simulink model "Commande_6_ReglageCascade_LoopShaping"  (R2015a)
settings: Solver=ode45  StartTime=0.0  StopTime=20  RelTol=1e-3
values from neighbouring files (symbols this model uses):
  Kd = p1^2*J4    (= 0.0333)    [A_1_Data.m]    (also in matlab.mat = 0.009)
  Kp = -2*p1*J4    (= 0.00222)    [A_1_Data.m]    (also in matlab.mat = 0.0006)
  s = tf('s')    [A_3_LoopShaping.m]    (also in A_4_Hinfini.m = zpk('s'))
  X = [0;0;0;0;0;0;0;0]    [A_1_Data.m]
  Y = [0;0;0;0;0;0;0;0]    [A_1_Data.m]
undefined symbols (not defined in the file or in its folder): sfun3d, Z
libraries: sm_lib x332, nesl_utility x15, simulink x1
(part 1 of 10)
settings Model: Creator=user  LastModifiedBy=user

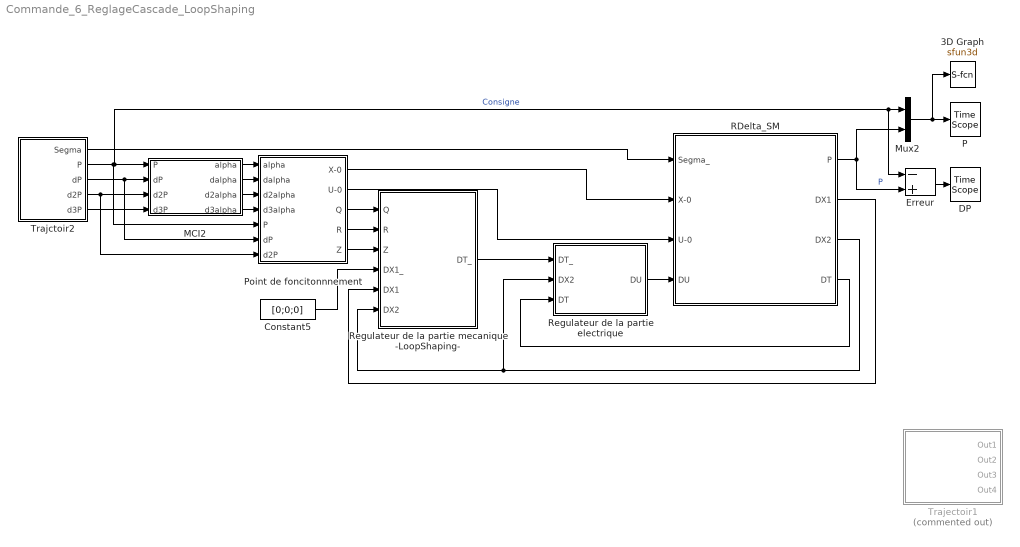
== system Commande_6_ReglageCascade_LoopShaping ==
  3D Graph : S-Function  LoadFcn=sfun3d([],[],[],'LoadBlock')  StartFcn=sfun3d([],[],[],'Start')  StopFcn=sfun3d([],[],[],'Stop')  FunctionName=sfun3d  Parameters=ax,T,np,cp,gd,ls,mk  mask(3D Graph){np=2, ax=[-1 1 -1 1 -2 0]*0.3, cp=[3 2 1], gd=on, ls=-, mk=o, T=0.0001}
      mask prompts: np "Number of point (lines)"; ax "[xmin xmax  ymin ymax zmin zmax]"; cp "Camera position (use [0 0 1] for 2D XY view)"; gd "Grid (on|off)"; ls "LineStyle"; mk "Marker"; T "Sampling Time"
      mask help:
      | This block plots the position of several points in the XYZ space. The input contains the coordinates of all the points (x1,y1,z1,x2,y2,z2,...).
      | The number of points (lines), the XYZ ranges, camera position, grid, linestyle, marker and sampling time, can be set as mask parameters.
      settings: CopyFcn=sfun3d([],[],[],'CopyBlock')  DeleteFcn=sfun3d([],[],[],'DeleteBlock')  NameChangeFcn=sfun3d([],[],[],'NameChange')
      mask Help:
      | This block plots the position of several points in the XYZ space. The input contains the coordinates of all the points (x1,y1,z1,x2,y2,z2,...).
      | The number of points (lines), the XYZ ranges, camera position, grid, linestyle, marker and sampling time, can be set as mask parameters.
      mask TypeOptions ls: - | -- | : | -. | none
      mask TypeOptions mk: none | . | + | o | * | x | square | diamond | v | ^ | > | < | pentagram | hexagram
      mask Display: plot([.05 .95 .95 .05 .05],[.45 .45 .95 .95 .45], 0.5+cos(0:0.1:2*pi)*0.3,0.7+sin(0:0.1:2*pi)*0.2)
  Constant5 : Constant  Value=[0;0;0]
  DP : TimeScope  DefaultConfigurationName=spbscopes.TimeScopeBlockCfg
  Erreur : Sum  Inputs=-+
  MCI2 : MATLAB Function  TreatAsAtomicUnit=on
  Mux2 : Mux  Inputs=2
  P : TimeScope  DefaultConfigurationName=spbscopes.TimeScopeBlockCfg
  Point de foncitonnnement : Subsystem
  RDelta_SM : Subsystem
      mask Display:
      | image(imread('DeltaImage2.PNG'))
      | port_label('input',1,'Segma')
      | port_label('input',2,'X-0')
      | port_label('input',3,'U-0')
      | port_label('input',4,'DU')
      | port_label('output',1,'P')
      | port_label('output',2,'DX1')
      | port_label('output',3,'DX2')
      | port_label('output',4,'DT')
  Regulateur de la partie electrique : Subsystem
  Regulateur de la partie mecanique -LoopShaping- : Subsystem
  Trajctoir2 : Subsystem
  Trajectoir1 : Subsystem  Commented=on
  wires:
  Trajctoir2/2(P) -> Erreur/1, Mux2/1, MCI2/1(P), Point de foncitonnnement/5(P)  "Consigne"
  Trajctoir2/3(dP) -> Point de foncitonnnement/6(dP), MCI2/2(dP)
  Trajctoir2/4(d2P) -> Point de foncitonnnement/7(d2P), MCI2/3(d2P)
  MCI2/3(d2alpha) -> Point de foncitonnnement/3(d2alpha)
  MCI2/2(dalpha) -> Point de foncitonnnement/2(dalpha)
  MCI2/1(alpha) -> Point de foncitonnnement/1(alpha)
  MCI2/4(d3alpha) -> Point de foncitonnnement/4(d3alpha)
  Trajctoir2/5(d3P) -> MCI2/4(d3P)
  RDelta_SM/1(P) -> Mux2/2, Erreur/2  "P"
  Point de foncitonnnement/3(Q) -> Regulateur de la partie mecanique -LoopShaping-/1(Q)
  Point de foncitonnnement/4(R) -> Regulateur de la partie mecanique -LoopShaping-/2(R)
  Point de foncitonnnement/5(Z) -> Regulateur de la partie mecanique -LoopShaping-/3(Z)
  Point de foncitonnnement/2(U-0) -> RDelta_SM/3(U-0)
  Point de foncitonnnement/1(X-0) -> RDelta_SM/2(X-0)
  Regulateur de la partie electrique/1(DU) -> RDelta_SM/4(DU)
  Regulateur de la partie mecanique -LoopShaping-/1(DT_) -> Regulateur de la partie electrique/1(DT_)
  RDelta_SM/4(DT) -> Regulateur de la partie electrique/3(DT)
  RDelta_SM/3(DX2) -> Regulateur de la partie mecanique -LoopShaping-/6(DX2), Regulateur de la partie electrique/2(DX2)
  RDelta_SM/2(DX1) -> Regulateur de la partie mecanique -LoopShaping-/5(DX1)
  Constant5/1 -> Regulateur de la partie mecanique -LoopShaping-/4(DX1_)
  Trajctoir2/1(Segma) -> RDelta_SM/1(Segma_)
  Mux2/1 -> 3D Graph/1, P/1
  Erreur/1 -> DP/1

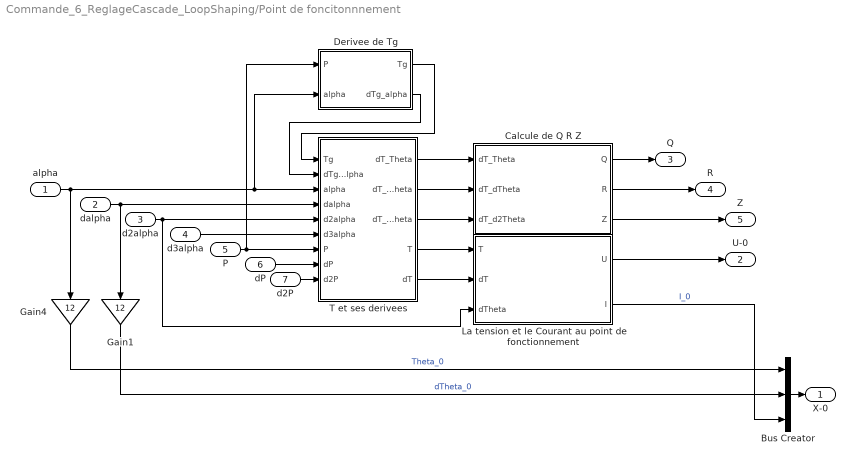
== system Commande_6_ReglageCascade_LoopShaping/Point de foncitonnnement ==
  alpha : Inport
  dalpha : Inport  Port=2
  d2alpha : Inport  Port=3
  d3alpha : Inport  Port=4
  P : Inport  Port=5
  dP : Inport  Port=6
  d2P : Inport  Port=7
  Bus Creator : BusCreator  Inputs=3
  "Calcule de Q R Z " : MATLAB Function  TreatAsAtomicUnit=on
  Derivee de Tg : Subsystem
  Gain1 : Gain  Gain=12
  Gain4 : Gain  Gain=12
  La tension et le Courant au point de fonctionnement : MATLAB Function  TreatAsAtomicUnit=on
  T et ses derivees : Subsystem
  X-0 : Outport
  U-0 : Outport  Port=2
  Q : Outport  Port=3
  R : Outport  Port=4
  Z : Outport  Port=5
  wires:
  alpha/1 -> Derivee de Tg/2(alpha), T et ses derivees/3(alpha), Gain4/1
  dalpha/1 -> Gain1/1, T et ses derivees/4(dalpha)
  P/1 -> Derivee de Tg/1(P), T et ses derivees/7(P)
  dP/1 -> T et ses derivees/8(dP)
  d2P/1 -> T et ses derivees/9(d2P)
  T et ses derivees/5(dT) -> La tension et le Courant au point de fonctionnement/2(dT)
  Derivee de Tg/2(dTg_alpha) -> T et ses derivees/2(dTg_alpha)
  Derivee de Tg/1(Tg) -> T et ses derivees/1(Tg)
  d3alpha/1 -> T et ses derivees/6(d3alpha)
  T et ses derivees/4(T) -> La tension et le Courant au point de fonctionnement/1(T)
  La tension et le Courant au point de fonctionnement/1(U) -> U-0/1
  Bus Creator/1 -> X-0/1
  Gain4/1 -> Bus Creator/1  "Theta_0"
  Gain1/1 -> Bus Creator/2  "dTheta_0"
  d2alpha/1 -> La tension et le Courant au point de fonctionnement/3(dTheta), T et ses derivees/5(d2alpha)
  La tension et le Courant au point de fonctionnement/2(I) -> Bus Creator/3  "I_0"
  "Calcule de Q R Z "/2(R) -> R/1
  "Calcule de Q R Z "/3(Z) -> Z/1
  "Calcule de Q R Z "/1(Q) -> Q/1
  T et ses derivees/2(dT_dTheta) -> "Calcule de Q R Z "/2(dT_dTheta)
  T et ses derivees/1(dT_Theta) -> "Calcule de Q R Z "/1(dT_Theta)
  T et ses derivees/3(dT_d2Theta) -> "Calcule de Q R Z "/3(dT_d2Theta)

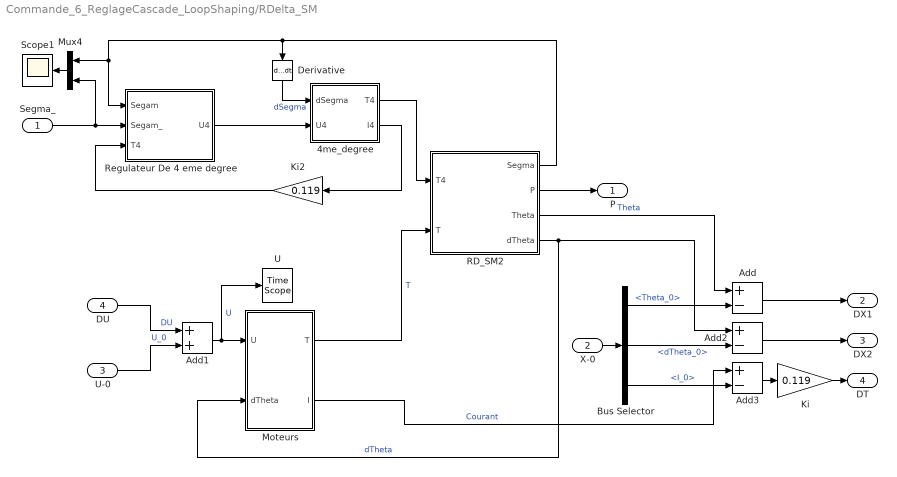
== system Commande_6_ReglageCascade_LoopShaping/RDelta_SM ==
  Segma_ : Inport
  X-0 : Inport  Port=2
  U-0 : Inport  Port=3
  DU : Inport  Port=4
  4me_degree : Subsystem
      mask Display:
      | image(imread('motor4.jpg'))
      | port_label('output',1,'T4')
      | port_label('output',2,'I4')
      | port_label('input',2,'U4')
      | port_label('input',1,'dSegma')
  Add : Sum  Inputs=+-
  Add1 : Sum
  Add2 : Sum  Inputs=+-
  Add3 : Sum  Inputs=+-
  Bus Selector : BusSelector  OutputSignals=Theta_0,dTheta_0,I_0
  Derivative : Derivative
  Ki : Gain  Gain=0.119
  Ki2 : Gain  Gain=0.119
  Moteurs : Subsystem
      mask Display:
      | image(imread('image_motor.jpg'))
      | port_label('output',1,'T')
      | port_label('output',2,'I')
      | port_label('input',1,'U')
      | port_label('input',2,'dTheta')
  Mux4 : Mux  Inputs=2
  RD_SM2 : Subsystem
      mask Display:
      | image(imread('DeltaImage2.PNG'))
      | port_label('input',1,'T4')
      | port_label('input',2,'T')
      | port_label('output',1,'Segma')
      | port_label('output',2,'P')
      | port_label('output',3,'Theta')
      | port_label('output',4,'dTheta')
  Regulateur De 4 eme degree : Subsystem
  Scope1 : Scope
      settings: YMin=-3.5  YMax=6.5  SaveName=ScopeData5
  U : TimeScope  DefaultConfigurationName=spbscopes.TimeScopeBlockCfg
  P : Outport
  DX1 : Outport  Port=2
  DX2 : Outport  Port=3
  DT : Outport  Port=4
  wires:
  Moteurs/2(I) -> Add3/1  "Courant"
  Add1/1 -> U/1, Moteurs/1(U)  "U"
  RD_SM2/3(Theta) -> Add/1  "Theta"
  RD_SM2/4(dTheta) -> Moteurs/2(dTheta), Add2/1  "dTheta"
  Moteurs/1(T) -> RD_SM2/2(T)  "T"
  RD_SM2/2(P) -> P/1
  Add/1 -> DX1/1
  DU/1 -> Add1/1  "DU"
  U-0/1 -> Add1/2  "U_0"
  X-0/1 -> Bus Selector/1
  Add2/1 -> DX2/1
  Add3/1 -> Ki/1
  Bus Selector/1 -> Add/2  "<Theta_0>"
  Bus Selector/2 -> Add2/2  "<dTheta_0>"
  Bus Selector/3 -> Add3/2  "<I_0>"
  Ki/1 -> DT/1
  RD_SM2/1(Segma) -> Derivative/1, Mux4/1, Regulateur De 4 eme degree/1(Segam)
  Derivative/1 -> 4me_degree/1(dSegma)  "dSegma"
  4me_degree/1(T4) -> RD_SM2/1(T4)
  Regulateur De 4 eme degree/1(U4) -> 4me_degree/2(U4)
  Ki2/1 -> Regulateur De 4 eme degree/3(T4)
  4me_degree/2(I4) -> Ki2/1
  Segma_/1 -> Mux4/2, Regulateur De 4 eme degree/2(Segam_)
  Mux4/1 -> Scope1/1

== system Commande_6_ReglageCascade_LoopShaping/Regulateur de la partie electrique ==
  DT_ : Inport
  DX2 : Inport  Port=2
  DT : Inport  Port=3
  Calcule de gains1 : MATLAB Function  TreatAsAtomicUnit=on
  Decoupleur Tension Vitess : MATLAB Function  TreatAsAtomicUnit=on
  Integrator2 : Integrator
  Sum1 : Sum  Inputs=|+-
  Sum2 : Sum  Inputs=+|+
  DU : Outport
  wires:
  Sum1/1 -> Calcule de gains1/1(e)  "e"
  Integrator2/1 -> Sum2/1
  Calcule de gains1/2(ep) -> Sum2/2
  Calcule de gains1/1(ei) -> Integrator2/1
  DT/1 -> Sum1/2
  DT_/1 -> Sum1/1
  Decoupleur Tension Vitess/1(DU) -> DU/1
  DX2/1 -> Decoupleur Tension Vitess/2(DX2)
  Sum2/1 -> Decoupleur Tension Vitess/1(DUd)  "DUd"

== system Commande_6_ReglageCascade_LoopShaping/Regulateur de la partie mecanique -LoopShaping- ==
  Q : Inport
  R : Inport  Port=2
  Z : Inport  Port=3
  DX1_ : Inport  Port=4
  DX1 : Inport  Port=5
  DX2 : Inport  Port=6
  Decoupleur1 : MATLAB Function  TreatAsAtomicUnit=on
  Demux : Demux  Outputs=3
  Mux : Mux  Inputs=3
  R LoopShaping : TransferFcn  Numerator="[70.7    1654.6]"  Denominator="[0.0047    1.0000]"
  R LoopShaping1 : TransferFcn  Numerator="[70.7    1654.6]"  Denominator="[0.0047    1.0000]"
  R LoopShaping2 : TransferFcn  Numerator="[70.7    1654.6]"  Denominator="[0.0047    1.0000]"
  RE : MATLAB Function  TreatAsAtomicUnit=on
  Sum12 : Sum  Inputs=|+-
  DT_ : Outport
  wires:
  DX1/1 -> Sum12/2, RE/4(DX1), Decoupleur1/5(DX1)
  Decoupleur1/1(DT_) -> DT_/1
  Q/1 -> Decoupleur1/1(Q), RE/1(Q)
  R/1 -> Decoupleur1/2(R), RE/2(R)
  Z/1 -> Decoupleur1/3(Z)
  DX2/1 -> Decoupleur1/6(DX2), RE/5(DX2)
  Sum12/1 -> Demux/1
  Mux/1 -> RE/3(E)
  DX1_/1 -> Sum12/1
  RE/1(V) -> Decoupleur1/4(V)
  Demux/1 -> R LoopShaping/1
  Demux/2 -> R LoopShaping1/1
  Demux/3 -> R LoopShaping2/1
  R LoopShaping/1 -> Mux/1
  R LoopShaping1/1 -> Mux/2
  R LoopShaping2/1 -> Mux/3

== system Commande_6_ReglageCascade_LoopShaping/Trajctoir2 ==
  Constant4 : Constant  Value=4
  Memory : Memory  X0=[ 0 ; 0]
  Memory1 : Memory  X0=13
  Memory2 : Memory  X0=3*pi/2/3 +2*pi/3
  Memory3 : Memory  X0=1
  Memory4 : Memory  X0=-pi
  Rotary Switch2 : Subsystem  DialogController=hmiCreateDDGDialog  IsWebBlock=on  mask(MathWorksWebBlock){webBlockId=84b7631a-e5b0-4c75-a53e-23700f43ee0a, webBlockType=discreteknob, ShowInLibBrowser=on, ShowInitialText=on, HMISrcModelName=[]}
      mask prompts: webBlockId "WebBlock Id"; webBlockType "WebBlock Type"; HMISrcModelName "Source Model"
      mask Help: helpview([docroot '/mapfiles/simulink.map'], 'hmi_rotary_switch')
      mask Display:
      | model = bdroot(gcb);
      | if strcmp(get_param(model,'BlockDiagramType'), 'library')
      |     image([(matlabroot) '/toolbox/simulink/hmi/icons/DiscreteKnob.png']);
      | end
  Trajectoir1 : MATLAB Function  TreatAsAtomicUnit=on
  Trajectoir2 : MATLAB Function  TreatAsAtomicUnit=on
  t1 : Clock
  Segma : Outport
  P : Outport  Port=2
  dP : Outport  Port=3
  d2P : Outport  Port=4
  d3P : Outport  Port=5
  wires:
  Trajectoir2/1(DPP) -> Memory/1
  Memory/1 -> Trajectoir2/1(DP)
  Memory1/1 -> Trajectoir2/2(i)
  Trajectoir2/2(ii) -> Memory1/1
  t1/1 -> Trajectoir2/11(t), Trajectoir1/2(t)
  Constant4/1 -> Trajectoir1/1(ne)
  Trajectoir1/2(P) -> Trajectoir2/7(P)
  Trajectoir1/3(dP) -> Trajectoir2/8(dP)
  Trajectoir1/4(d2P) -> Trajectoir2/9(d2P)
  Trajectoir1/5(d3P) -> Trajectoir2/10(d3P)
  Memory2/1 -> Trajectoir2/3(t0)
  Trajectoir2/3(tt0) -> Memory2/1
  Trajectoir2/7(P_) -> P/1
  Trajectoir2/8(dP_) -> dP/1
  Trajectoir2/9(d2P_) -> d2P/1
  Trajectoir2/10(d3P_) -> d3P/1
  Memory3/1 -> Trajectoir2/4(n)
  Trajectoir2/4(nn) -> Memory3/1
  Memory4/1 -> Trajectoir2/5(S)
  Trajectoir2/5(SS) -> Memory4/1
  Trajectoir1/1(Segma) -> Trajectoir2/6(Segma)
  Trajectoir2/6(Segma_) -> Segma/1

== system Commande_6_ReglageCascade_LoopShaping/Trajectoir1 ==
  Clock2 : Clock
  Constant3 : Constant  Value=4
  Rotary Switch1 : Subsystem  DialogController=hmiCreateDDGDialog  IsWebBlock=on  mask(MathWorksWebBlock){webBlockId=1c237f34-4d4e-4242-8d80-e82ed52eea22, webBlockType=discreteknob, ShowInLibBrowser=on, ShowInitialText=on, HMISrcModelName=[]}
      mask prompts: webBlockId "WebBlock Id"; webBlockType "WebBlock Type"; HMISrcModelName "Source Model"
      mask Help: helpview([docroot '/mapfiles/simulink.map'], 'hmi_rotary_switch')
      mask Display:
      | model = bdroot(gcb);
      | if strcmp(get_param(model,'BlockDiagramType'), 'library')
      |     image([(matlabroot) '/toolbox/simulink/hmi/icons/DiscreteKnob.png']);
      | end
  Trajectoir2 : MATLAB Function  TreatAsAtomicUnit=on
  Out1 : Outport
  Out2 : Outport  Port=2
  Out3 : Outport  Port=3
  Out4 : Outport  Port=4
  wires:
  Constant3/1 -> Trajectoir2/2(ne)
  Clock2/1 -> Trajectoir2/1(t)
  Trajectoir2/3(d2P) -> Out3/1
  Trajectoir2/1(P) -> Out1/1
  Trajectoir2/2(dP) -> Out2/1
  Trajectoir2/4(d3P) -> Out4/1

== system Commande_6_ReglageCascade_LoopShaping/Point de foncitonnnement/Derivee de Tg ==
  P : Inport
  alpha : Inport  Port=2
  Gravite_lineaire : MATLAB Function  TreatAsAtomicUnit=on
  Jinv : MATLAB Function  TreatAsAtomicUnit=on
  Tg : Outport
  dTg_alpha : Outport  Port=2
  wires:
  P/1 -> Jinv/1(P), Gravite_lineaire/1(P)
  alpha/1 -> Gravite_lineaire/2(alpha)
  Jinv/1(Jinv) -> Gravite_lineaire/3(Jinv)
  Gravite_lineaire/2(dTg_Theta) -> dTg_alpha/1
  Gravite_lineaire/1(Tg) -> Tg/1

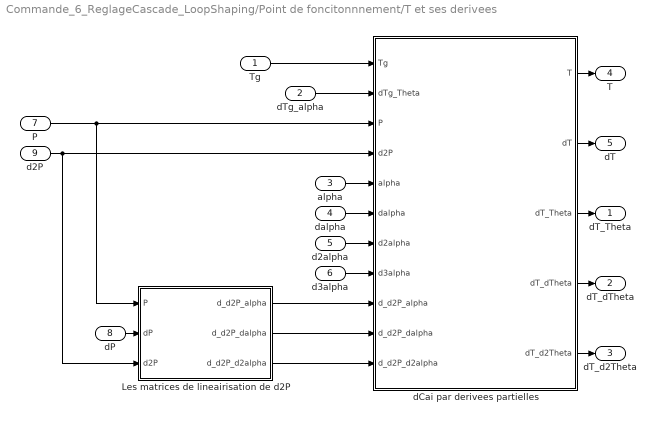
== system Commande_6_ReglageCascade_LoopShaping/Point de foncitonnnement/T et ses derivees ==
  Tg : Inport
  dTg_alpha : Inport  Port=2
  alpha : Inport  Port=3
  dalpha : Inport  Port=4
  d2alpha : Inport  Port=5
  d3alpha : Inport  Port=6
  P : Inport  Port=7
  dP : Inport  Port=8
  d2P : Inport  Port=9
  "Les matrices de lineairisation de d2P  " : MATLAB Function  TreatAsAtomicUnit=on
  "dCai par derivees partielles " : MATLAB Function  TreatAsAtomicUnit=on
  dT_Theta : Outport
  dT_dTheta : Outport  Port=2
  dT_d2Theta : Outport  Port=3
  T : Outport  Port=4
  dT : Outport  Port=5
  wires:
  "Les matrices de lineairisation de d2P  "/2(d_d2P_dalpha) -> "dCai par derivees partielles "/10(d_d2P_dalpha)
  "Les matrices de lineairisation de d2P  "/3(d_d2P_d2alpha) -> "dCai par derivees partielles "/11(d_d2P_d2alpha)
  "Les matrices de lineairisation de d2P  "/1(d_d2P_alpha) -> "dCai par derivees partielles "/9(d_d2P_alpha)
  P/1 -> "Les matrices de lineairisation de d2P  "/1(P), "dCai par derivees partielles "/3(P)
  d2P/1 -> "Les matrices de lineairisation de d2P  "/3(d2P), "dCai par derivees partielles "/4(d2P)
  alpha/1 -> "dCai par derivees partielles "/5(alpha)
  dalpha/1 -> "dCai par derivees partielles "/6(dalpha)
  d2alpha/1 -> "dCai par derivees partielles "/7(d2alpha)
  dP/1 -> "Les matrices de lineairisation de d2P  "/2(dP)
  "dCai par derivees partielles "/3(dT_Theta) -> dT_Theta/1
  "dCai par derivees partielles "/4(dT_dTheta) -> dT_dTheta/1
  "dCai par derivees partielles "/5(dT_d2Theta) -> dT_d2Theta/1
  dTg_alpha/1 -> "dCai par derivees partielles "/2(dTg_Theta)
  Tg/1 -> "dCai par derivees partielles "/1(Tg)
  d3alpha/1 -> "dCai par derivees partielles "/8(d3alpha)
  "dCai par derivees partielles "/1(T) -> T/1
  "dCai par derivees partielles "/2(dT) -> dT/1

== system Commande_6_ReglageCascade_LoopShaping/RDelta_SM/4me_degree ==
  dSegma : Inport
  U4 : Inport  Port=2
  Integrator : Integrator
  Ki : Gain  Gain=0.119
  equations electriques : MATLAB Function  TreatAsAtomicUnit=on
  T4 : Outport
  I4 : Outport  Port=2
  wires:
  Ki/1 -> T4/1  "T"
  dSegma/1 -> equations electriques/3(dTheta)
  equations electriques/1(dI) -> Integrator/1  "dI"
  Integrator/1 -> equations electriques/1(I), Ki/1, I4/1  "I"
  U4/1 -> equations electriques/2(U)

== system Commande_6_ReglageCascade_LoopShaping/RDelta_SM/Moteurs ==
  U : Inport
  dTheta : Inport  Port=2
  Integrator : Integrator  InitialCondition=-0.1041*[1;1;1]
  Ki : Gain  Gain=0.119
  Scope13 : Scope
      settings: TimeRange=0.507510643892459  YMin=-1000  YMax=1000  SaveName=ScopeData24
  equations electriques : MATLAB Function  TreatAsAtomicUnit=on
  T : Outport
  I : Outport  Port=2
  wires:
  U/1 -> equations electriques/2(U)
  Integrator/1 -> I/1, Scope13/1, Ki/1, equations electriques/1(I)  "I"
  equations electriques/1(dI) -> Integrator/1  "dI"
  dTheta/1 -> equations electriques/3(dTheta)
  Ki/1 -> T/1  "T"

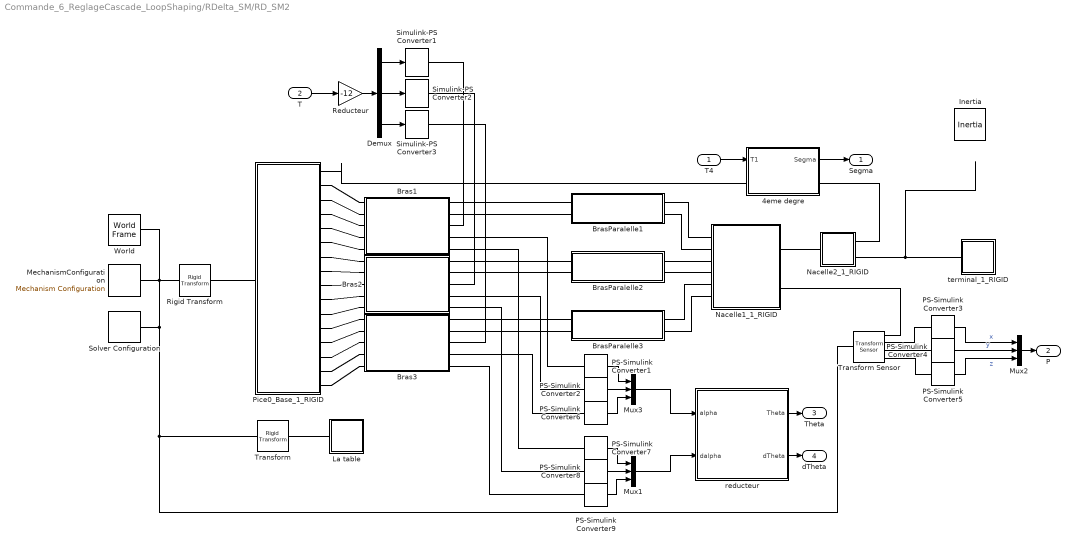
== system Commande_6_ReglageCascade_LoopShaping/RDelta_SM/RD_SM2 ==
  T4 : Inport
  T : Inport  Port=2
  4eme degre : Subsystem
  Bras1 : Subsystem
  Bras2 : Subsystem
  Bras3 : Subsystem
  BrasParalelle1 : Subsystem
  BrasParalelle2 : Subsystem
  BrasParalelle3 : Subsystem
  Demux : Demux  Outputs=3
  Inertia : sm_lib/Body Elements/Inertia  InertiaType=PointMass  Mass=20  MassUnits=kg  CenterOfMass=[0 0 0]  CenterOfMassUnits=m  MomentsOfInertia=[1 1 1]  MomentsOfInertiaUnits=kg*m^2  ProductsOfInertia=[0 0 0]  ProductsOfInertiaUnits=kg*m^2  BlockFunction=simmechanics.library.body_elements.inertia
  La table : Subsystem
  MechanismConfiguration : sm_lib/Utilities/Mechanism Configuration  UniformGravity=Constant  GravityVector=[0 0 -9.98]  GravityUnits=m/s^2  LinearizationDelta=0.001  BlockFunction=simmechanics.library.utilities.mechanism_configuration
  Mux1 : Mux  Inputs=3
  Mux2 : Mux  Inputs=3
  Mux3 : Mux  Inputs=3
  Nacelle1_1_RIGID : Subsystem
  Nacelle2_1_RIGID : Subsystem
  PS-Simulink Converter1 : nesl_utility/PS-Simulink Converter  PhysicalDomain=network_engine_domain  SubClassName=ps_output  LeftPortType=input  RightPortType=output  PseudoPeriodic=off  Frequencies=[]  Unit=rad  AffineConversion=off
  PS-Simulink Converter2 : nesl_utility/PS-Simulink Converter  PhysicalDomain=network_engine_domain  SubClassName=ps_output  LeftPortType=input  RightPortType=output  PseudoPeriodic=off  Frequencies=[]  Unit=rad  AffineConversion=off
  PS-Simulink Converter3 : nesl_utility/PS-Simulink Converter  PhysicalDomain=network_engine_domain  SubClassName=ps_output  LeftPortType=input  RightPortType=output  PseudoPeriodic=off  Frequencies=[]  Unit=m  AffineConversion=off
  PS-Simulink Converter4 : nesl_utility/PS-Simulink Converter  PhysicalDomain=network_engine_domain  SubClassName=ps_output  LeftPortType=input  RightPortType=output  PseudoPeriodic=off  Frequencies=[]  Unit=m  AffineConversion=off
  PS-Simulink Converter5 : nesl_utility/PS-Simulink Converter  PhysicalDomain=network_engine_domain  SubClassName=ps_output  LeftPortType=input  RightPortType=output  PseudoPeriodic=off  Frequencies=[]  Unit=m  AffineConversion=off
  PS-Simulink Converter6 : nesl_utility/PS-Simulink Converter  PhysicalDomain=network_engine_domain  SubClassName=ps_output  LeftPortType=input  RightPortType=output  PseudoPeriodic=off  Frequencies=[]  Unit=rad  AffineConversion=off
  PS-Simulink Converter7 : nesl_utility/PS-Simulink Converter  PhysicalDomain=network_engine_domain  SubClassName=ps_output  LeftPortType=input  RightPortType=output  PseudoPeriodic=off  Frequencies=[]  Unit=rad/s  AffineConversion=off
  PS-Simulink Converter8 : nesl_utility/PS-Simulink Converter  PhysicalDomain=network_engine_domain  SubClassName=ps_output  LeftPortType=input  RightPortType=output  PseudoPeriodic=off  Frequencies=[]  Unit=rad/s  AffineConversion=off
  PS-Simulink Converter9 : nesl_utility/PS-Simulink Converter  PhysicalDomain=network_engine_domain  SubClassName=ps_output  LeftPortType=input  RightPortType=output  PseudoPeriodic=off  Frequencies=[]  Unit=rad/s  AffineConversion=off
  Pice0_Base_1_RIGID : Subsystem
  Reducteur : Gain  Gain=-12
  Rigid Transform : sm_lib/Frames and Transforms/Rigid Transform  TranslationMethod=Cartesian  TranslationLengthUnit=mm  TranslationStandardAxis=+Z  TranslationStandardOffset=0  TranslationCartesianOffset=[0 0 115]  TranslationROffset=0  TranslationROffsetUnits=m  TranslationZOffset=0  TranslationZOffsetUnits=m  TranslationThetaOffset=0  TranslationThetaOffsetUnits=deg  RotationMethod=None  RotationAngleUnits=deg  RotationStandardAxis=+Z  RotationAngle=0.0  RotationArbitraryAxis=[0 0 1]  FollAlignAxisA=+X  BaseAlignAxisA=+Y  FollAlignAxisB=+Y  BaseAlignAxisB=+Z  RotationMatrix=[1 0 0; 0 1 0; 0 0 1]  BlockFunction=simmechanics.library.frames_transforms.rigid_transform
  Simulink-PS Converter1 : nesl_utility/Simulink-PS Converter  PhysicalDomain=network_engine_domain  SubClassName=ps_input  LeftPortType=input  RightPortType=output  PseudoPeriodic=off  Frequencies=[]  NoiseDistribution=none  NoiseParameters=[]  Unit=1  AffineConversion=off  InputFiltering=off  SimscapeFilterOrder=1  InputFilterTimeConstant=0.001  UdotUserProvided=1
  Simulink-PS Converter2 : nesl_utility/Simulink-PS Converter  PhysicalDomain=network_engine_domain  SubClassName=ps_input  LeftPortType=input  RightPortType=output  PseudoPeriodic=off  Frequencies=[]  NoiseDistribution=none  NoiseParameters=[]  Unit=1  AffineConversion=off  InputFiltering=off  SimscapeFilterOrder=1  InputFilterTimeConstant=0.001  UdotUserProvided=1
  Simulink-PS Converter3 : nesl_utility/Simulink-PS Converter  PhysicalDomain=network_engine_domain  SubClassName=ps_input  LeftPortType=input  RightPortType=output  PseudoPeriodic=off  Frequencies=[]  NoiseDistribution=none  NoiseParameters=[]  Unit=1  AffineConversion=off  InputFiltering=off  SimscapeFilterOrder=1  InputFilterTimeConstant=0.001  UdotUserProvided=1
  Solver Configuration : nesl_utility/Solver Configuration  PhysicalDomain=network_engine_domain  SubClassName=solver  LeftPortType=input  RightPortType=generic  Accelerate=off  Tones=[]  Harmonics=[]  SimulateNoise=off  Profile=off  UseLocalSampling=off  EnableSwitchedLinearOptims=on  FrequencyDomain=off  UseCCode=off  RelTol=0.001  AbsTol=1e-06  MinStep=1e-09  ToWorkspace=off  RevertToSquareIcSolve=off  NumHomotopyIterations=100  DoDC=off  ResidualTolerance=1e-09  UseLocalSolver=off  LocalSolverChoice=NE_BACKWARD_EULER_ADVANCER  LocalSolverSampleTime=0.001  DoFixedCost=off  MaxNonlinIter=3  MaxModeIter=2  LinearAlgebra=Sparse  DelaysMemoryBudget=1024  AutomaticFiltering=on  FilteringTimeConstant=0.001
  Transform : sm_lib/Frames and Transforms/Rigid Transform  TranslationMethod=Cartesian  TranslationLengthUnit=mm  TranslationStandardAxis=+Z  TranslationStandardOffset=0  TranslationCartesianOffset=[0 0 -388]  TranslationROffset=0  TranslationROffsetUnits=m  TranslationZOffset=0  TranslationZOffsetUnits=m  TranslationThetaOffset=0  TranslationThetaOffsetUnits=deg  RotationMethod=None  RotationAngleUnits=deg  RotationStandardAxis=+Z  RotationAngle=0.0  RotationArbitraryAxis=[0 0 1]  FollAlignAxisA=+X  BaseAlignAxisA=+Y  FollAlignAxisB=+Y  BaseAlignAxisB=+Z  RotationMatrix=[1 0 0; 0 1 0; 0 0 1]  BlockFunction=simmechanics.library.frames_transforms.rigid_transform
  Transform Sensor : sm_lib/Frames and Transforms/Transform Sensor  MeasurementFrame=World  SenseAngle=off  SenseAxis=off  SenseAngle1=off  SenseAngle2=off  SenseAngle3=off  SenseQ=off  SenseR=off  SenseOmegaX=off  SenseOmegaY=off  SenseOmegaZ=off  SenseOmega1=off  SenseOmega2=off  SenseOmega3=off  SenseQDot=off  SenseRDot=off  SenseAlphaX=off  SenseAlphaY=off  SenseAlphaZ=off  SenseAlpha1=off  SenseAlpha2=off  SenseAlpha3=off  SenseQDDot=off  SenseRDDot=off  SenseX=on  SenseY=on  SenseZ=on  SenseRad=off  SenseAzim=off  SenseDist=off  SenseInc=off  SenseXDot=off  SenseYDot=off  SenseZDot=off  SenseRadDot=off  SenseAzimDot=off  SenseDistDot=off  SenseIncDot=off  SenseXDDot=off  SenseYDDot=off  SenseZDDot=off  SenseRadDDot=off  SenseAzimDDot=off  SenseDistDDot=off  SenseIncDDot=off  BlockFunction=simmechanics.library.frames_transforms.transform_sensor
  World : sm_lib/Frames and Transforms/World Frame  BlockFunction=simmechanics.library.frames_transforms.world_frame
  reducteur : MATLAB Function  TreatAsAtomicUnit=on
  terminal_1_RIGID : Subsystem
  Segma : Outport
  P : Outport  Port=2
  Theta : Outport  Port=3
  dTheta : Outport  Port=4
  wires:
  PS-Simulink Converter5/1 -> Mux2/3  "z"
  PS-Simulink Converter3/1 -> Mux2/1  "x"
  PS-Simulink Converter4/1 -> Mux2/2  "y"
  Mux2/1 -> P/1
  Demux/1 -> Simulink-PS Converter1/1
  Demux/2 -> Simulink-PS Converter2/1
  T/1 -> Reducteur/1
  Reducteur/1 -> Demux/1
  Demux/3 -> Simulink-PS Converter3/1
  PS-Simulink Converter6/1 -> Mux3/3
  PS-Simulink Converter1/1 -> Mux3/1
  PS-Simulink Converter2/1 -> Mux3/2
  reducteur/1(Theta) -> Theta/1
  PS-Simulink Converter9/1 -> Mux1/3
  PS-Simulink Converter7/1 -> Mux1/1
  PS-Simulink Converter8/1 -> Mux1/2
  reducteur/2(dTheta) -> dTheta/1
  Mux3/1 -> reducteur/1(alpha)
  Mux1/1 -> reducteur/2(dalpha)
  4eme degre/1(Segma) -> Segma/1
  T4/1 -> 4eme degre/1(T1)
  connections:
  Bras1/RConn2 -- BrasParalelle1/LConn2
  Pice0_Base_1_RIGID/RConn3 -- Bras1/LConn2
  Pice0_Base_1_RIGID/RConn4 -- Bras1/LConn3
  Pice0_Base_1_RIGID/RConn5 -- Bras1/LConn4
  Pice0_Base_1_RIGID/RConn2 -- Bras1/LConn1
  Pice0_Base_1_RIGID/RConn6 -- Bras1/LConn5
  Bras1/RConn1 -- BrasParalelle1/LConn1
  Transform Sensor/RConn1 -- Nacelle1_1_RIGID/RConn2
  Transform Sensor/RConn2 -- PS-Simulink Converter3/LConn1
  PS-Simulink Converter5/LConn1 -- Transform Sensor/RConn4
  Rigid Transform/RConn1 -- Pice0_Base_1_RIGID/LConn1
  Nacelle2_1_RIGID/LConn1 -- Nacelle1_1_RIGID/RConn1
  Nacelle2_1_RIGID/RConn2 -- terminal_1_RIGID/LConn1
  Nacelle2_1_RIGID/RConn1 -- 4eme degre/RConn1
  Pice0_Base_1_RIGID/RConn1 -- 4eme degre/LConn1
  PS-Simulink Converter4/LConn1 -- Transform Sensor/RConn3
  Rigid Transform/LConn1 -- MechanismConfiguration/RConn1 -- World/RConn1 -- Transform/LConn1 -- Transform Sensor/LConn1 -- Solver Configuration/RConn1
  Bras2/RConn2 -- BrasParalelle2/LConn2
  BrasParalelle2/LConn1 -- Bras2/RConn1
  Bras3/RConn2 -- BrasParalelle3/LConn2
  BrasParalelle3/LConn1 -- Bras3/RConn1
  BrasParalelle1/RConn1 -- Nacelle1_1_RIGID/LConn1
  BrasParalelle1/RConn2 -- Nacelle1_1_RIGID/LConn2
  BrasParalelle2/RConn1 -- Nacelle1_1_RIGID/LConn3
  BrasParalelle2/RConn2 -- Nacelle1_1_RIGID/LConn4
  BrasParalelle3/RConn1 -- Nacelle1_1_RIGID/LConn5
  BrasParalelle3/RConn2 -- Nacelle1_1_RIGID/LConn6
  Pice0_Base_1_RIGID/RConn7 -- Bras2/LConn1
  Pice0_Base_1_RIGID/RConn8 -- Bras2/LConn2
  Pice0_Base_1_RIGID/RConn10 -- Bras2/LConn4
  Pice0_Base_1_RIGID/RConn9 -- Bras2/LConn3
  Pice0_Base_1_RIGID/RConn11 -- Bras2/LConn5
  Pice0_Base_1_RIGID/RConn16 -- Bras3/LConn5
  Pice0_Base_1_RIGID/RConn15 -- Bras3/LConn4
  Pice0_Base_1_RIGID/RConn14 -- Bras3/LConn3
  Pice0_Base_1_RIGID/RConn13 -- Bras3/LConn2
  Pice0_Base_1_RIGID/RConn12 -- Bras3/LConn1
  Bras1/RConn3 -- Simulink-PS Converter1/RConn1
  Bras2/RConn3 -- Simulink-PS Converter2/RConn1
  Bras3/RConn3 -- Simulink-PS Converter3/RConn1
  PS-Simulink Converter1/LConn1 -- Bras1/RConn4
  PS-Simulink Converter2/LConn1 -- Bras2/RConn4
  PS-Simulink Converter6/LConn1 -- Bras3/RConn4
  PS-Simulink Converter7/LConn1 -- Bras1/RConn5
  PS-Simulink Converter8/LConn1 -- Bras2/RConn5
  PS-Simulink Converter9/LConn1 -- Bras3/RConn5
  La table/LConn1 -- Transform/RConn1

== system Commande_6_ReglageCascade_LoopShaping/RDelta_SM/Regulateur De 4 eme degree ==
  Segam : Inport
  Segam_ : Inport  Port=2
  T4 : Inport  Port=3
  Add6 : Sum  Inputs=-+
  Derivative : Derivative
  PID Controller : simulink/Continuous/PID Controller  Controller=PID  TimeDomain=Continuous-time  SampleTime=-1  IntegratorMethod=Forward Euler  FilterMethod=Forward Euler  Form=Parallel  UseFilter=on  ControllerParametersSource=internal  P=Kp  I=0  D=Kd  N=100  InitialConditionSource=internal  InitialConditionForIntegrator=0  InitialConditionForFilter=0  ExternalReset=none  LimitOutput=off  UpperSaturationLimit=inf  LowerSaturationLimit=-inf  LinearizeAsGain=on  AntiWindupMode=none  Kb=1  TrackingMode=off  Kt=1  PParamMin=[]  PParamMax=[]  IParamMin=[]  IParamMax=[]  DParamMin=[]  DParamMax=[]  NParamMin=[]  NParamMax=[]  KbParamMin=[]  KbParamMax=[]  KtParamMin=[]  KtParamMax=[]  POutMin=[]  POutMax=[]  IOutMin=[]  IOutMax=[]  DOutMin=[]  DOutMax=[]  NOutMin=[]  NOutMax=[]  KbOutMin=[]  KbOutMax=[]  KtOutMin=[]  KtOutMax=[]  IntegratorOutMin=[]  IntegratorOutMax=[]  FilterOutMin=[]  FilterOutMax=[]  SumOutMin=[]  SumOutMax=[]  SumI1OutMin=[]  SumI1OutMax=[]  SumI2OutMin=[]  SumI2OutMax=[]  SumI3OutMin=[]  SumI3OutMax=[]  SumDOutMin=[]  SumDOutMax=[]  SaturationOutMin=[]  SaturationOutMax=[]  IntegratorContinuousStateAttributes=''  IntegratorStateMustResolveToSignalObject=off  IntegratorRTWStateStorageClass=Auto  FilterContinuousStateAttributes=''  FilterStateMustResolveToSignalObject=off  FilterRTWStateStorageClass=Auto  DifferentiatorICPrevScaledInput=0  DifferentiatorOutMin=[]  DifferentiatorOutMax=[]
  Regulateur: Tension_Couple : Subsystem
  U4 : Outport
  wires:
  PID Controller/1 -> Regulateur: Tension_Couple/2(T4_)
  Add6/1 -> PID Controller/1
  Segam/1 -> Add6/1, Derivative/1
  Segam_/1 -> Add6/2
  Derivative/1 -> Regulateur: Tension_Couple/1(dSegma)
  T4/1 -> Regulateur: Tension_Couple/3(T4)
  Regulateur: Tension_Couple/1(U4) -> U4/1

== system Commande_6_ReglageCascade_LoopShaping/Trajctoir2/Rotary Switch2 ==

== system Commande_6_ReglageCascade_LoopShaping/Trajectoir1/Rotary Switch1 ==

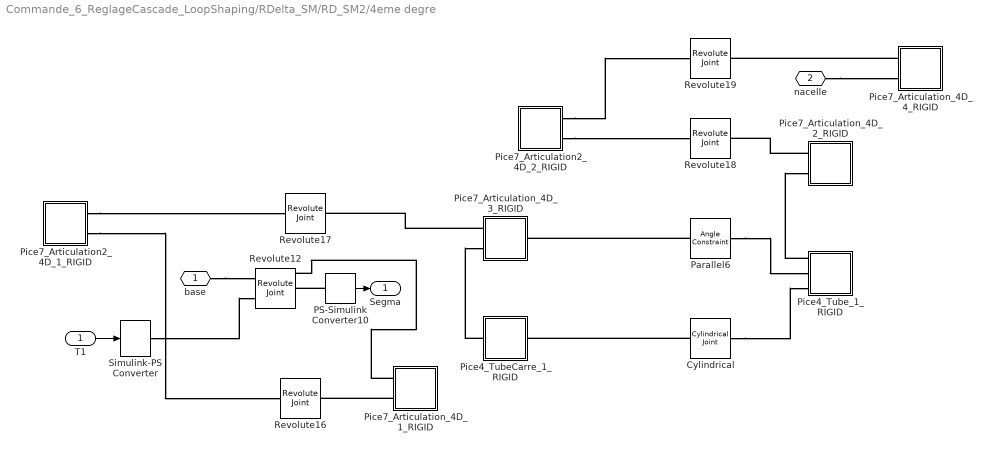
== system Commande_6_ReglageCascade_LoopShaping/RDelta_SM/RD_SM2/4eme degre ==
  T1 : Inport
  Cylindrical : sm_lib/Joints/Cylindrical Joint  SenseConstraintForce=off  SenseConstraintForceX=off  SenseConstraintForceY=off  SenseConstraintForceZ=off  SenseConstraintTorque=off  SenseConstraintTorqueX=off  SenseConstraintTorqueY=off  SenseConstraintTorqueZ=off  SenseTotalForce=off  SenseTotalForceX=off  SenseTotalForceY=off  SenseTotalForceZ=off  SenseTotalTorque=off  SenseTotalTorqueX=off  SenseTotalTorqueY=off  SenseTotalTorqueZ=off  CompositeWrenchDir=FollowerOnBase  CompositeWrenchFrame=BaseFrame  PzEquilibriumPosition=0  PzEquilibriumPositionUnits=m  PzSpringStiffness=0  PzSpringStiffnessUnits=N/m  PzDampingCoefficient=0  PzDampingCoefficientUnits=s*N/m  PzTorqueActuationMode=NoTorque  PzMotionActuationMode=ComputedMotion  PzSensePosition=off  PzSenseVelocity=off  PzSenseAcceleration=off  PzSenseTorqueForce=off  PzPositionTargetSpecify=on  PzPositionTargetPriority=Low  PzPositionTargetValue=0  PzPositionTargetValueUnits=mm  PzVelocityTargetSpecify=off  PzVelocityTargetPriority=High  PzVelocityTargetValue=0  PzVelocityTargetValueUnits=m/s  RzEquilibriumPosition=0  RzEquilibriumPositionUnits=rad  RzSpringStiffness=0  RzSpringStiffnessUnits=m*N/rad  RzDampingCoefficient=0  RzDampingCoefficientUnits=m*s*N/rad  RzTorqueActuationMode=NoTorque  RzMotionActuationMode=ComputedMotion  RzSensePosition=off  RzSenseVelocity=off  RzSenseAcceleration=off  RzSenseTorqueForce=off  RzPositionTargetSpecify=on  RzPositionTargetPriority=Low  RzPositionTargetValue=90  RzPositionTargetValueUnits=deg  RzVelocityTargetSpecify=off  RzVelocityTargetPriority=High  RzVelocityTargetValue=0  RzVelocityTargetValueUnits=deg/s  BlockFunction=simmechanics.library.joints.cylindrical_joint
  PS-Simulink Converter10 : nesl_utility/PS-Simulink Converter  PhysicalDomain=network_engine_domain  SubClassName=ps_output  LeftPortType=input  RightPortType=output  PseudoPeriodic=off  Frequencies=[]  Unit=rad  AffineConversion=off
  Parallel6 : sm_lib/Constraints/Angle Constraint  ConstraintType=Parallel  Angle=45  AngleUnits=deg  SenseSignedTorqueMagnitude=off  SenseTorque=off  SenseForce=off  WrenchDir=FollowerOnBase  WrenchFrame=BaseFrame  BlockFunction=simmechanics.library.constraints.angle_constraint
  Pice4_TubeCarre_1_RIGID : Subsystem
  Pice4_Tube_1_RIGID : Subsystem
  Pice7_Articulation2_4D_1_RIGID : Subsystem
  Pice7_Articulation2_4D_2_RIGID : Subsystem
  Pice7_Articulation_4D_1_RIGID : Subsystem
  Pice7_Articulation_4D_2_RIGID : Subsystem
  Pice7_Articulation_4D_3_RIGID : Subsystem
  Pice7_Articulation_4D_4_RIGID : Subsystem
  Revolute12 : sm_lib/Joints/Revolute Joint  SenseConstraintForce=off  SenseConstraintForceX=off  SenseConstraintForceY=off  SenseConstraintForceZ=off  SenseConstraintTorque=off  SenseConstraintTorqueX=off  SenseConstraintTorqueY=off  SenseConstraintTorqueZ=off  SenseTotalForce=off  SenseTotalForceX=off  SenseTotalForceY=off  SenseTotalForceZ=off  SenseTotalTorque=off  SenseTotalTorqueX=off  SenseTotalTorqueY=off  SenseTotalTorqueZ=off  CompositeWrenchDir=FollowerOnBase  CompositeWrenchFrame=BaseFrame  EquilibriumPosition=0  EquilibriumPositionUnits=rad  SpringStiffness=0  SpringStiffnessUnits=m*N/rad  DampingCoefficient=0  DampingCoefficientUnits=m*s*N/rad  TorqueActuationMode=InputTorque  MotionActuationMode=ComputedMotion  SensePosition=on  SenseVelocity=on  SenseAcceleration=off  SenseTorqueForce=off  PositionTargetSpecify=on  PositionTargetPriority=Low  PositionTargetValue=0  PositionTargetValueUnits=deg  VelocityTargetSpecify=off  VelocityTargetPriority=High  VelocityTargetValue=0  VelocityTargetValueUnits=deg/s  BlockFunction=simmechanics.library.joints.revolute_joint
  Revolute16 : sm_lib/Joints/Revolute Joint  SenseConstraintForce=off  SenseConstraintForceX=off  SenseConstraintForceY=off  SenseConstraintForceZ=off  SenseConstraintTorque=off  SenseConstraintTorqueX=off  SenseConstraintTorqueY=off  SenseConstraintTorqueZ=off  SenseTotalForce=off  SenseTotalForceX=off  SenseTotalForceY=off  SenseTotalForceZ=off  SenseTotalTorque=off  SenseTotalTorqueX=off  SenseTotalTorqueY=off  SenseTotalTorqueZ=off  CompositeWrenchDir=FollowerOnBase  CompositeWrenchFrame=BaseFrame  EquilibriumPosition=0  EquilibriumPositionUnits=rad  SpringStiffness=0  SpringStiffnessUnits=m*N/rad  DampingCoefficient=0  DampingCoefficientUnits=m*s*N/rad  TorqueActuationMode=NoTorque  MotionActuationMode=ComputedMotion  SensePosition=off  SenseVelocity=off  SenseAcceleration=off  SenseTorqueForce=off  PositionTargetSpecify=off  PositionTargetPriority=Low  PositionTargetValue=90.000000000000071  PositionTargetValueUnits=deg  VelocityTargetSpecify=off  VelocityTargetPriority=High  VelocityTargetValue=0  VelocityTargetValueUnits=deg/s  BlockFunction=simmechanics.library.joints.revolute_joint
  Revolute17 : sm_lib/Joints/Revolute Joint  SenseConstraintForce=off  SenseConstraintForceX=off  SenseConstraintForceY=off  SenseConstraintForceZ=off  SenseConstraintTorque=off  SenseConstraintTorqueX=off  SenseConstraintTorqueY=off  SenseConstraintTorqueZ=off  SenseTotalForce=off  SenseTotalForceX=off  SenseTotalForceY=off  SenseTotalForceZ=off  SenseTotalTorque=off  SenseTotalTorqueX=off  SenseTotalTorqueY=off  SenseTotalTorqueZ=off  CompositeWrenchDir=FollowerOnBase  CompositeWrenchFrame=BaseFrame  EquilibriumPosition=0  EquilibriumPositionUnits=rad  SpringStiffness=0  SpringStiffnessUnits=m*N/rad  DampingCoefficient=0  DampingCoefficientUnits=m*s*N/rad  TorqueActuationMode=NoTorque  MotionActuationMode=ComputedMotion  SensePosition=off  SenseVelocity=off  SenseAcceleration=off  SenseTorqueForce=off  PositionTargetSpecify=off  PositionTargetPriority=Low  PositionTargetValue=180  PositionTargetValueUnits=deg  VelocityTargetSpecify=off  VelocityTargetPriority=High  VelocityTargetValue=0  VelocityTargetValueUnits=deg/s  BlockFunction=simmechanics.library.joints.revolute_joint
  Revolute18 : sm_lib/Joints/Revolute Joint  SenseConstraintForce=off  SenseConstraintForceX=off  SenseConstraintForceY=off  SenseConstraintForceZ=off  SenseConstraintTorque=off  SenseConstraintTorqueX=off  SenseConstraintTorqueY=off  SenseConstraintTorqueZ=off  SenseTotalForce=off  SenseTotalForceX=off  SenseTotalForceY=off  SenseTotalForceZ=off  SenseTotalTorque=off  SenseTotalTorqueX=off  SenseTotalTorqueY=off  SenseTotalTorqueZ=off  CompositeWrenchDir=FollowerOnBase  CompositeWrenchFrame=BaseFrame  EquilibriumPosition=0  EquilibriumPositionUnits=rad  SpringStiffness=0  SpringStiffnessUnits=m*N/rad  DampingCoefficient=0  DampingCoefficientUnits=m*s*N/rad  TorqueActuationMode=NoTorque  MotionActuationMode=ComputedMotion  SensePosition=off  SenseVelocity=off  SenseAcceleration=off  SenseTorqueForce=off  PositionTargetSpecify=off  PositionTargetPriority=Low  PositionTargetValue=2.2657964386729655e-13  PositionTargetValueUnits=deg  VelocityTargetSpecify=off  VelocityTargetPriority=High  VelocityTargetValue=0  VelocityTargetValueUnits=deg/s  BlockFunction=simmechanics.library.joints.revolute_joint
  Revolute19 : sm_lib/Joints/Revolute Joint  SenseConstraintForce=off  SenseConstraintForceX=off  SenseConstraintForceY=off  SenseConstraintForceZ=off  SenseConstraintTorque=off  SenseConstraintTorqueX=off  SenseConstraintTorqueY=off  SenseConstraintTorqueZ=off  SenseTotalForce=off  SenseTotalForceX=off  SenseTotalForceY=off  SenseTotalForceZ=off  SenseTotalTorque=off  SenseTotalTorqueX=off  SenseTotalTorqueY=off  SenseTotalTorqueZ=off  CompositeWrenchDir=FollowerOnBase  CompositeWrenchFrame=BaseFrame  EquilibriumPosition=0  EquilibriumPositionUnits=rad  SpringStiffness=0  SpringStiffnessUnits=m*N/rad  DampingCoefficient=0  DampingCoefficientUnits=m*s*N/rad  TorqueActuationMode=NoTorque  MotionActuationMode=ComputedMotion  SensePosition=off  SenseVelocity=off  SenseAcceleration=off  SenseTorqueForce=off  PositionTargetSpecify=off  PositionTargetPriority=Low  PositionTargetValue=89.999999999999588  PositionTargetValueUnits=deg  VelocityTargetSpecify=off  VelocityTargetPriority=High  VelocityTargetValue=0  VelocityTargetValueUnits=deg/s  BlockFunction=simmechanics.library.joints.revolute_joint
  Simulink-PS Converter : nesl_utility/Simulink-PS Converter  PhysicalDomain=network_engine_domain  SubClassName=ps_input  LeftPortType=input  RightPortType=output  PseudoPeriodic=off  Frequencies=[]  NoiseDistribution=none  NoiseParameters=[]  Unit=1  AffineConversion=off  InputFiltering=off  SimscapeFilterOrder=1  InputFilterTimeConstant=0.001  UdotUserProvided=1
  base : PMIOPort  Port=1  Side=Left
  nacelle : PMIOPort  Port=2  Side=Right
  Segma : Outport
  wires:
  PS-Simulink Converter10/1 -> Segma/1
  T1/1 -> Simulink-PS Converter/1
  connections:
  base/RConn1 -- Revolute12/LConn1
  Pice7_Articulation_4D_1_RIGID/LConn1 -- Revolute12/RConn1
  Pice4_TubeCarre_1_RIGID/LConn1 -- Pice7_Articulation_4D_3_RIGID/LConn2
  Pice7_Articulation2_4D_1_RIGID/RConn2 -- Revolute16/LConn1
  Pice7_Articulation_4D_1_RIGID/LConn2 -- Revolute16/RConn1
  Pice7_Articulation2_4D_1_RIGID/RConn1 -- Revolute17/LConn1
  Pice7_Articulation_4D_3_RIGID/LConn1 -- Revolute17/RConn1
  Pice7_Articulation2_4D_2_RIGID/RConn2 -- Revolute18/LConn1
  Pice7_Articulation_4D_2_RIGID/LConn1 -- Revolute18/RConn1
  Pice7_Articulation2_4D_2_RIGID/RConn1 -- Revolute19/LConn1
  Pice7_Articulation_4D_4_RIGID/LConn1 -- Revolute19/RConn1
  nacelle/RConn1 -- Pice7_Articulation_4D_4_RIGID/LConn2
  Cylindrical/LConn1 -- Pice4_TubeCarre_1_RIGID/RConn1
  Cylindrical/RConn1 -- Pice4_Tube_1_RIGID/LConn3
  Pice4_Tube_1_RIGID/LConn1 -- Pice7_Articulation_4D_2_RIGID/LConn2
  Parallel6/LConn1 -- Pice7_Articulation_4D_3_RIGID/RConn1
  Parallel6/RConn1 -- Pice4_Tube_1_RIGID/LConn2
  Simulink-PS Converter/RConn1 -- Revolute12/LConn2
  PS-Simulink Converter10/LConn1 -- Revolute12/RConn2

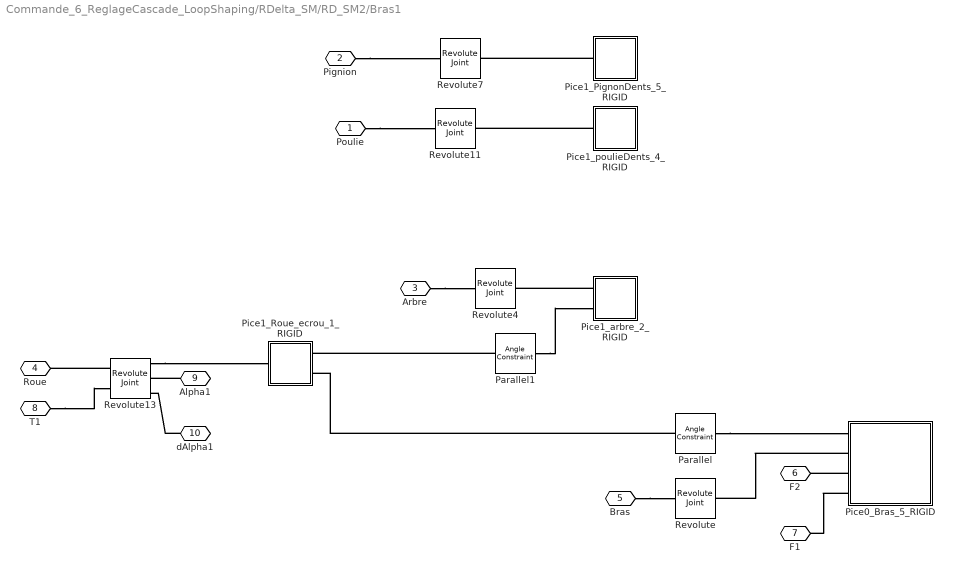
== system Commande_6_ReglageCascade_LoopShaping/RDelta_SM/RD_SM2/Bras1 ==
  Parallel : sm_lib/Constraints/Angle Constraint  ConstraintType=Parallel  Angle=45  AngleUnits=deg  SenseSignedTorqueMagnitude=off  SenseTorque=off  SenseForce=off  WrenchDir=FollowerOnBase  WrenchFrame=BaseFrame  BlockFunction=simmechanics.library.constraints.angle_constraint
  Parallel1 : sm_lib/Constraints/Angle Constraint  ConstraintType=Parallel  Angle=45  AngleUnits=deg  SenseSignedTorqueMagnitude=off  SenseTorque=off  SenseForce=off  WrenchDir=FollowerOnBase  WrenchFrame=BaseFrame  BlockFunction=simmechanics.library.constraints.angle_constraint
  Pice0_Bras_5_RIGID : Subsystem
  Pice1_PignonDents_5_RIGID : Subsystem
  Pice1_Roue_ecrou_1_RIGID : Subsystem
  Pice1_arbre_2_RIGID : Subsystem
  Pice1_poulieDents_4_RIGID : Subsystem
  Revolute : sm_lib/Joints/Revolute Joint  SenseConstraintForce=off  SenseConstraintForceX=off  SenseConstraintForceY=off  SenseConstraintForceZ=off  SenseConstraintTorque=off  SenseConstraintTorqueX=off  SenseConstraintTorqueY=off  SenseConstraintTorqueZ=off  SenseTotalForce=off  SenseTotalForceX=off  SenseTotalForceY=off  SenseTotalForceZ=off  SenseTotalTorque=off  SenseTotalTorqueX=off  SenseTotalTorqueY=off  SenseTotalTorqueZ=off  CompositeWrenchDir=FollowerOnBase  CompositeWrenchFrame=BaseFrame  EquilibriumPosition=0  EquilibriumPositionUnits=rad  SpringStiffness=0  SpringStiffnessUnits=m*N/rad  DampingCoefficient=0  DampingCoefficientUnits=m*s*N/rad  TorqueActuationMode=NoTorque  MotionActuationMode=ComputedMotion  SensePosition=off  SenseVelocity=off  SenseAcceleration=off  SenseTorqueForce=off  PositionTargetSpecify=on  PositionTargetPriority=Low  PositionTargetValue=67.987395610882629  PositionTargetValueUnits=deg  VelocityTargetSpecify=off  VelocityTargetPriority=High  VelocityTargetValue=0  VelocityTargetValueUnits=deg/s  BlockFunction=simmechanics.library.joints.revolute_joint
  Revolute11 : sm_lib/Joints/Revolute Joint  SenseConstraintForce=off  SenseConstraintForceX=off  SenseConstraintForceY=off  SenseConstraintForceZ=off  SenseConstraintTorque=off  SenseConstraintTorqueX=off  SenseConstraintTorqueY=off  SenseConstraintTorqueZ=off  SenseTotalForce=off  SenseTotalForceX=off  SenseTotalForceY=off  SenseTotalForceZ=off  SenseTotalTorque=off  SenseTotalTorqueX=off  SenseTotalTorqueY=off  SenseTotalTorqueZ=off  CompositeWrenchDir=FollowerOnBase  CompositeWrenchFrame=BaseFrame  EquilibriumPosition=0  EquilibriumPositionUnits=rad  SpringStiffness=0  SpringStiffnessUnits=m*N/rad  DampingCoefficient=0  DampingCoefficientUnits=m*s*N/rad  TorqueActuationMode=NoTorque  MotionActuationMode=ComputedMotion  SensePosition=off  SenseVelocity=off  SenseAcceleration=off  SenseTorqueForce=off  PositionTargetSpecify=on  PositionTargetPriority=Low  PositionTargetValue=-180  PositionTargetValueUnits=deg  VelocityTargetSpecify=off  VelocityTargetPriority=High  VelocityTargetValue=0  VelocityTargetValueUnits=deg/s  BlockFunction=simmechanics.library.joints.revolute_joint
  Revolute13 : sm_lib/Joints/Revolute Joint  SenseConstraintForce=off  SenseConstraintForceX=off  SenseConstraintForceY=off  SenseConstraintForceZ=off  SenseConstraintTorque=off  SenseConstraintTorqueX=off  SenseConstraintTorqueY=off  SenseConstraintTorqueZ=off  SenseTotalForce=off  SenseTotalForceX=off  SenseTotalForceY=off  SenseTotalForceZ=off  SenseTotalTorque=off  SenseTotalTorqueX=off  SenseTotalTorqueY=off  SenseTotalTorqueZ=off  CompositeWrenchDir=FollowerOnBase  CompositeWrenchFrame=BaseFrame  EquilibriumPosition=0  EquilibriumPositionUnits=rad  SpringStiffness=0  SpringStiffnessUnits=m*N/rad  DampingCoefficient=0  DampingCoefficientUnits=m*s*N/rad  TorqueActuationMode=InputTorque  MotionActuationMode=ComputedMotion  SensePosition=on  SenseVelocity=on  SenseAcceleration=off  SenseTorqueForce=off  PositionTargetSpecify=on  PositionTargetPriority=Low  PositionTargetValue=-112.01260438911736  PositionTargetValueUnits=deg  VelocityTargetSpecify=off  VelocityTargetPriority=High  VelocityTargetValue=0  VelocityTargetValueUnits=deg/s  BlockFunction=simmechanics.library.joints.revolute_joint
  Revolute4 : sm_lib/Joints/Revolute Joint  SenseConstraintForce=off  SenseConstraintForceX=off  SenseConstraintForceY=off  SenseConstraintForceZ=off  SenseConstraintTorque=off  SenseConstraintTorqueX=off  SenseConstraintTorqueY=off  SenseConstraintTorqueZ=off  SenseTotalForce=off  SenseTotalForceX=off  SenseTotalForceY=off  SenseTotalForceZ=off  SenseTotalTorque=off  SenseTotalTorqueX=off  SenseTotalTorqueY=off  SenseTotalTorqueZ=off  CompositeWrenchDir=FollowerOnBase  CompositeWrenchFrame=BaseFrame  EquilibriumPosition=0  EquilibriumPositionUnits=rad  SpringStiffness=0  SpringStiffnessUnits=m*N/rad  DampingCoefficient=0  DampingCoefficientUnits=m*s*N/rad  TorqueActuationMode=NoTorque  MotionActuationMode=ComputedMotion  SensePosition=off  SenseVelocity=off  SenseAcceleration=off  SenseTorqueForce=off  PositionTargetSpecify=on  PositionTargetPriority=Low  PositionTargetValue=-112.01260438911737  PositionTargetValueUnits=deg  VelocityTargetSpecify=off  VelocityTargetPriority=High  VelocityTargetValue=0  VelocityTargetValueUnits=deg/s  BlockFunction=simmechanics.library.joints.revolute_joint
  Revolute7 : sm_lib/Joints/Revolute Joint  SenseConstraintForce=off  SenseConstraintForceX=off  SenseConstraintForceY=off  SenseConstraintForceZ=off  SenseConstraintTorque=off  SenseConstraintTorqueX=off  SenseConstraintTorqueY=off  SenseConstraintTorqueZ=off  SenseTotalForce=off  SenseTotalForceX=off  SenseTotalForceY=off  SenseTotalForceZ=off  SenseTotalTorque=off  SenseTotalTorqueX=off  SenseTotalTorqueY=off  SenseTotalTorqueZ=off  CompositeWrenchDir=FollowerOnBase  CompositeWrenchFrame=BaseFrame  EquilibriumPosition=0  EquilibriumPositionUnits=rad  SpringStiffness=0  SpringStiffnessUnits=m*N/rad  DampingCoefficient=0  DampingCoefficientUnits=m*s*N/rad  TorqueActuationMode=NoTorque  MotionActuationMode=ComputedMotion  SensePosition=off  SenseVelocity=off  SenseAcceleration=off  SenseTorqueForce=off  PositionTargetSpecify=on  PositionTargetPriority=Low  PositionTargetValue=-180  PositionTargetValueUnits=deg  VelocityTargetSpecify=off  VelocityTargetPriority=High  VelocityTargetValue=0  VelocityTargetValueUnits=deg/s  BlockFunction=simmechanics.library.joints.revolute_joint
  Poulie : PMIOPort  Port=1  Side=Left
  Pignion : PMIOPort  Port=2  Side=Left
  Arbre : PMIOPort  Port=3  Side=Left
  Roue : PMIOPort  Port=4  Side=Left
  Bras : PMIOPort  Port=5  Side=Left
  F2 : PMIOPort  Port=6  Side=Right
  F1 : PMIOPort  Port=7  Side=Right
  T1 : PMIOPort  Port=8  Side=Right
  Alpha1 : PMIOPort  Port=9  Side=Right
  dAlpha1 : PMIOPort  Port=10  Side=Right
  connections:
  Bras/RConn1 -- Revolute/LConn1
  Pice1_arbre_2_RIGID/LConn1 -- Revolute4/RConn1
  Pignion/RConn1 -- Revolute7/LConn1
  Pice1_PignonDents_5_RIGID/LConn1 -- Revolute7/RConn1
  Pice0_Bras_5_RIGID/LConn2 -- Revolute/RConn1
  Poulie/RConn1 -- Revolute11/LConn1
  Pice1_poulieDents_4_RIGID/LConn1 -- Revolute11/RConn1
  Pice0_Bras_5_RIGID/LConn4 -- F1/RConn1
  Pice0_Bras_5_RIGID/LConn3 -- F2/RConn1
  Revolute13/LConn1 -- Roue/RConn1
  Revolute13/RConn1 -- Pice1_Roue_ecrou_1_RIGID/LConn1
  Parallel/LConn1 -- Pice1_Roue_ecrou_1_RIGID/RConn2
  Parallel/RConn1 -- Pice0_Bras_5_RIGID/LConn1
  Parallel1/LConn1 -- Pice1_Roue_ecrou_1_RIGID/RConn1
  Parallel1/RConn1 -- Pice1_arbre_2_RIGID/LConn2
  Arbre/RConn1 -- Revolute4/LConn1
  T1/RConn1 -- Revolute13/LConn2
  Alpha1/RConn1 -- Revolute13/RConn2
  dAlpha1/RConn1 -- Revolute13/RConn3
